simulink model "UNO_GenericOneWire_task"  (Simulink 3.00)
libraries: mathlib x5, REXduino_library x4, genlib x1, arclib x1

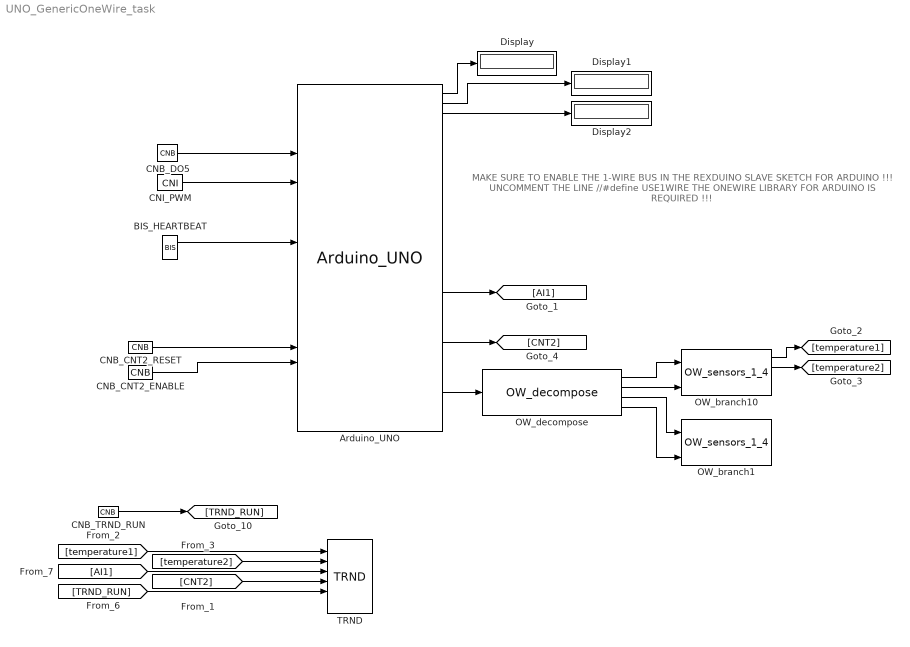
== system UNO_GenericOneWire_task ==
  note: MAKE SURE TO ENABLE THE 1-WIRE BUS IN
      | THE REXDUINO SLAVE SKETCH FOR ARDUINO !!!
      |
      | UNCOMMENT THE LINE //#define USE1WIRE
      | THE ONEWIRE LIBRARY FOR ARDUINO IS REQUIRED !!!
  Arduino_UNO : REXduino_library/Arduino_UNO  comPort=/dev/ttyACM0  pinmode2=8: Counter  pinmode3=1: Not connected  pinmode4=10: Counter DIR / Encoder B  pinmode5=2: Digital output  pinmode6=1: Not connected  pinmode9=5: PWM (analog output)  pinmode10=7: 1-Wire temperature  pinmode11=7: 1-Wire temperature  pinmodeA0=6: Analog input  pinmodeA1=1: Not connected  pinmodeA2=1: Not connected  pinmodeA3=1: Not connected  pinmodeA4=1: Not connected  pinmodeA5=1: Not connected  usercmd=1: No data
  BIS_HEARTBEAT : genlib/BIS  Y0=off  t1=0.7  t2=0.8  t3=0.9  t4=1.0  t5=0  t6=6  t7=7  t8=8  RPT=on  bEdit=off
  CNB_CNT2_ENABLE : mathlib/CNB  YCN=on
  CNB_CNT2_RESET : mathlib/CNB  YCN=off
  CNB_DO5 : mathlib/CNB  YCN=on
  CNB_TRND_RUN : mathlib/CNB  YCN=on
  CNI_PWM : mathlib/CNI  icn=128
  Display : Display
      settings: Format=Best fit
  Display1 : Display
      settings: Format=Best fit
  Display2 : Display
      settings: Format=Best fit
  OW_branch1 : REXduino_library/OW_sensors_1_4
      mask Type: REX sequence
  OW_branch10 : REXduino_library/OW_sensors_1_4
      mask Type: REX sequence
  OW_decompose : REXduino_library/OW_decompose
      mask Type: REX sequence
  TRND : arclib/TRND  n=4  l=1000  btype=8: Double  ptype1=1: Store  ptype2=1: Store  ptype3=1: Store  ptype4=1: Store  pfac=1  afac=0  arc=0  id=1  Title=Data trend  timesrc=1
  wires:
  Arduino_UNO/1 -> Display/1
  Arduino_UNO/2 -> Display1/1
  Arduino_UNO/3 -> Display2/1
  Arduino_UNO/21 -> [AI1]
  Arduino_UNO/26 -> [CNT2]
  Arduino_UNO/31 -> OW_decompose/1
  BIS_HEARTBEAT/1 -> Arduino_UNO/10
  CNB_CNT2_ENABLE/1 -> Arduino_UNO/18
  CNB_CNT2_RESET/1 -> Arduino_UNO/17
  CNB_DO5/1 -> Arduino_UNO/4
  CNB_TRND_RUN/1 -> [TRND_RUN]
  CNI_PWM/1 -> Arduino_UNO/6
  [CNT2] -> TRND/4
  [temperature1] -> TRND/1
  [temperature2] -> TRND/2
  [TRND_RUN] -> TRND/5
  [AI1] -> TRND/3
  OW_branch10/1 -> [temperature1]
  OW_branch10/2 -> [temperature2]
  OW_decompose/1 -> OW_branch10/1
  OW_decompose/2 -> OW_branch10/2
  OW_decompose/3 -> OW_branch1/1
  OW_decompose/4 -> OW_branch1/2
